simulink model "sgMdl_FaultInsertionControl"  (R2024b)
settings: Solver=FixedStepAuto  StartTime=0.0  StopTime=inf  RelTol=1e-3  EnableMultiTasking=on
libraries: simulink x1, speedgoatlib_PIL x1
Description:
  | Fault Insertion Control
settings Model: ModifiedByFormat=Speedgoat  SimulationMode=external  ExtModeTrigDuration=100000  Creator=Speedgoat  LastModifiedBy=Speedgoat
settings SolverCC: ConcurrentTasks=on  AlgebraicLoopSolver=TrustRegion  PositivePriorityOrder=on  InsertRTBMode=Never (minimum delay)
settings DataIOCC: SaveFormat=Array  SaveState=on  SignalLoggingName=logsOut
settings OptimizationCC: BlockReduction=off  BooleanDataType=off  OptimizeBlockIOStorage=off  BufferReuse=off  ReuseModelBlockBuffer=off  GlobalBufferReuse=off  ExpressionFolding=off  LocalBlockOutputs=off  InitFltsAndDblsToZero=on  OptimizeDataStoreBuffers=off  BusAssignmentInplaceUpdate=off
settings DebuggingCC: SaveWithParameterizedLinksMsg=none  UnderspecifiedInitializationDetection=Classic  MergeDetectMultiDrivingBlocksExec=none  CheckExecutionContextPreStartOutputMsg=on  SignalResolutionControl=TryResolveAllWithWarning  TasksWithSamePriorityMsg=none  UnconnectedInputMsg=warning  UnconnectedOutputMsg=warning  UnconnectedLineMsg=warning  SFUnexpectedBacktrackingDiag=warning  SFNoUnconditionalDefaultTransitionDiag=warning  SFExecutionAtInitializationDiag=none  ArithmeticOperatorsInVariantConditions=warning
settings HardwareCC: ProdBitPerLong=64  ProdLongLongMode=on  ProdHWDeviceType=Intel->x86-64 (Linux 64)
settings ModelReferenceCC: EnableRefExpFcnMdlSchedulingChecks=on  PropagateSignalLabelsOutOfModel=off
settings SFSimCC: SimUseLocalCustomCode=off  SimTargetLang=C++
settings RTWCC: Description=Speedgoat Real-Time Target Machine  SystemTargetFile=speedgoat.tlc  TemplateMakefile=slrealtime_default_tmf  PostCodeGenCommand=sg.model.build.makeCfg(bdroot, buildInfo);  RTWUseLocalCustomCode=off  Toolchain=Simulink Real-Time Toolchain  BuildConfiguration=Faster Runs  TargetLang=C++  GPUComputeCapability=3.5  DLArmComputeVersion=19.05
settings CodeAppCC: StateflowObjectComments=on
settings SimulinkRealTimeTargetCC: SubcomponentCodeInterfacePackaging=Reusable function  MATLABClassNameForMDSCustomization=Simulink.SoftwareTarget.GRTCustomization  InstructionSetFMA=off  LogToMDFFile=off  SLRTFileLogMaxRuns=10  UseGCCFastMath=on
settings ConfigComp: CovMetricSettings=dw  CovSaveCumulativeToWorkspaceVar=on  CovSaveSingleToWorkspaceVar=on  CovExternalEMLEnable=off  CovSFcnEnable=off  CovBoundaryAbsTol=1.0e-5

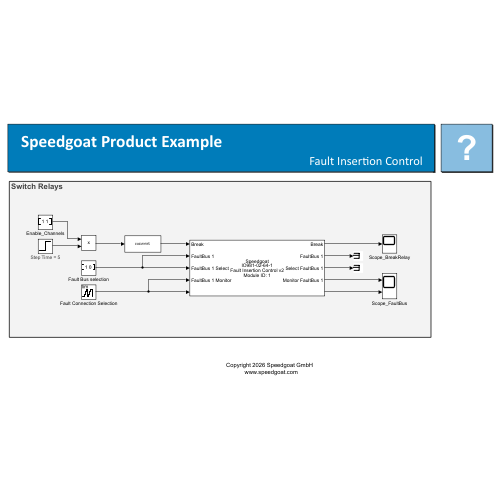
[thumbnail: Simulink's stored preview of the top-level diagram]
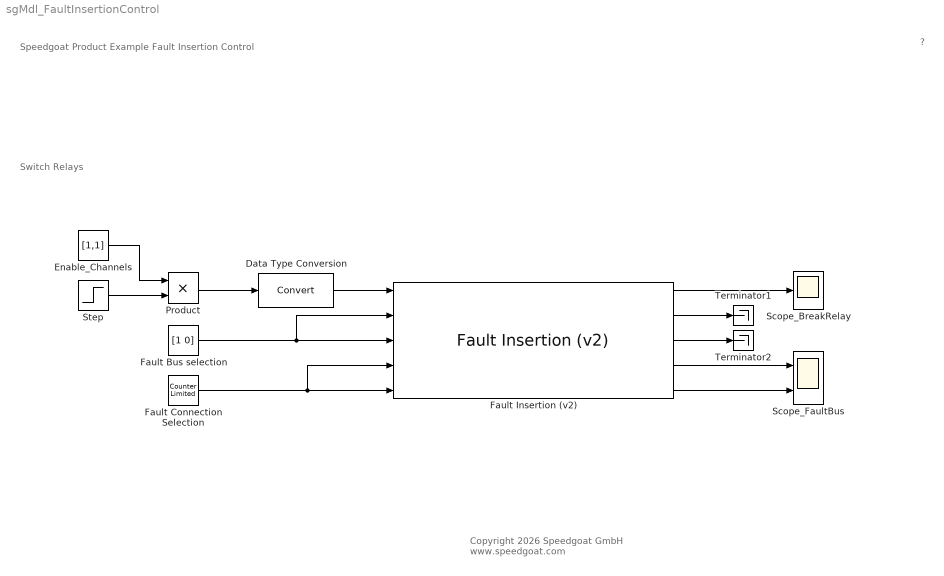
== system sgMdl_FaultInsertionControl ==
  note: Switch Relays
  note: Speedgoat Product Example
      | Fault Insertion Control
  note: ?
  note: Copyright 2026 Speedgoat GmbH
      |  www.speedgoat.com
  Data Type Conversion : DataTypeConversion  SaturateOnIntegerOverflow=off  RndMeth=Floor
  Enable_Channels : Constant  Value=[1,1]  SampleTime=1
  Fault Bus selection : Constant  Value=[1 0]  OutDataTypeStr=Inherit: Inherit via back propagation  SampleTime=1
  Fault Connection Selection : simulink/Sources/Counter Limited  uplimit=3  tsamp=1
  "Fault Insertion (v2) " : speedgoatlib_PIL/Fault Insertion (v2)   id=1  card_type="IO983-02-75-2  (2A Fault Insertion Switch, 75 channels, 2 fault buses)"  channel_vector=[1,2]  init_vector_break=[0]  init_vector_fault1=[0]  init_vector_fault2=[0]  reset_vector_break=[1]  reset_vector_fault1=[1]  reset_vector_fault2=[1]  show_output=on  ts=-1  slot=-1  NumCh=75  NumFB=2  NumFperMux=3  NumMperMux=0  NumMux=2  DeviceID=0  SubDeviceID=0  VendorID=0
      settings: SourceProductName=Simulink Real-Time: Speedgoat I/O Blockset
  Product : Product  OutDataTypeStr=Inherit: Inherit via back propagation
  Scope_BreakRelay : Scope
  Scope_FaultBus : Scope  NumInputPorts=2
  Step : Step  Time=5  SampleTime=1
      settings: AttributesFormatString=Step Time = %<Time>
  Terminator1 : Terminator
  Terminator2 : Terminator
  wires:
  Product/1 -> Data Type Conversion/1
  Enable_Channels/1 -> Product/1
  Step/1 -> Product/2
  Data Type Conversion/1 -> "Fault Insertion (v2) "/1
  Fault Connection Selection/1 -> "Fault Insertion (v2) "/5, "Fault Insertion (v2) "/4
  Fault Bus selection/1 -> "Fault Insertion (v2) "/3, "Fault Insertion (v2) "/2
  "Fault Insertion (v2) "/1 -> Scope_BreakRelay/1
  "Fault Insertion (v2) "/2 -> Terminator1/1
  "Fault Insertion (v2) "/3 -> Terminator2/1
  "Fault Insertion (v2) "/4 -> Scope_FaultBus/1
  "Fault Insertion (v2) "/5 -> Scope_FaultBus/2
